simulink subsystem "Controller"  (R2020a)
settings: Solver=VariableStepAuto  StartTime=0.0  StopTime=10.0  RelTol=1e-3
undefined symbols (not defined in the file): N, PWM, TMAX, tmax, TMIN, tmin, Ts, Ui, Xi
libraries: mpclib x1
settings Model: Creator=Lamarre  LastModifiedBy=lamarre

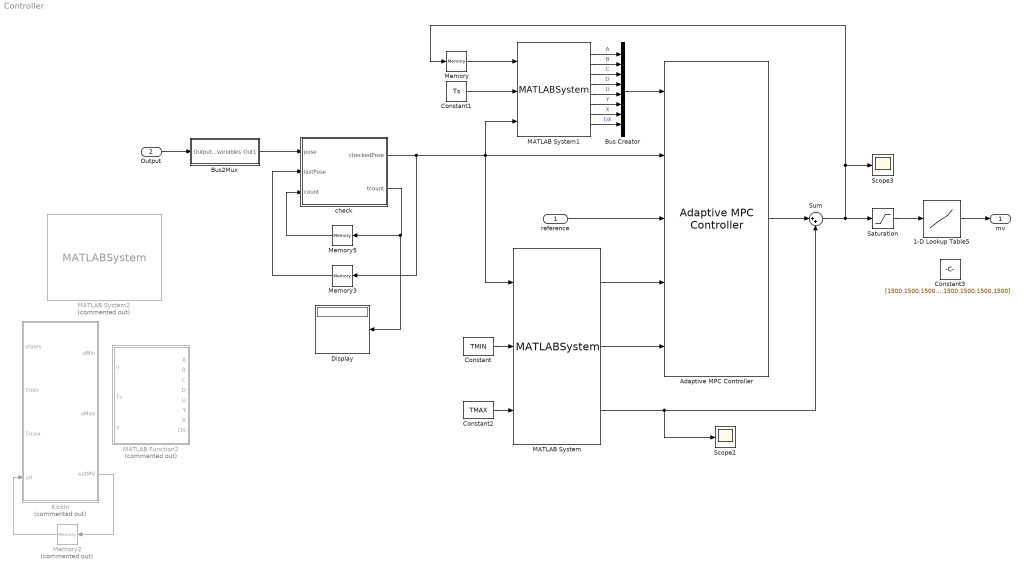
== system Controller ==
  reference : Inport
  Output : Inport  Port=2
  1-D Lookup Table5 : Lookup_n-D  NumberOfTableDimensions=1  BreakpointsForDimension1=N  Table=PWM  InterpMethod=Nearest  ExtrapMethod=Clip  InternalRulePriority=Speed  RndMeth=Simplest  InputSameDT=on
  Adaptive MPC Controller : mpclib/Adaptive MPC Controller  SCDEnableBlockLinearizationSpecification=on  mpcobj=mpcobj  enable_value=0  updateMPCinCallerWorkspace=on  md_inport=off  mv_inport=off  uref_inport=off  return_cost=off  return_mvseq=off  return_qpstatus=off  return_xseq=off  return_state=off  return_ovseq=off  state_inport=off  isltv_plant=off  umin_inport=on  umax_inport=on  ymin_inport=off  ymax_inport=off  cc_inport=off  ywt_inport=off  uwt_inport=off  duwt_inport=off  rhoeps_inport=off  pm_inport=off  MaximumP=10  HorizonChoice=FixedHorizon  BlockDataType=double  SampleTimeInherited=off  switch_inport=off
  Bus Creator : BusCreator  Inputs=8
  Bus2Mux : Subsystem
  Constant : Constant  Value=TMIN  VectorParams1D=off
  Constant1 : Constant  Value=Ts
  Constant2 : Constant  Value=TMAX
  Constant3 : Constant  Value=[1500,1500,1500,1500,1500,1500,1500,1500]
  Display : Display
  KickIn : MATLAB Function  Commented=on  TreatAsAtomicUnit=on  SystemSampleTime=Ts
  MATLAB Function2 : MATLAB Function  Commented=on  TreatAsAtomicUnit=on  SystemSampleTime=Ts
  MATLAB System : MATLABSystem  System=KickIn  SimulateUsing=Code generation
      mask Type: KickIn
      mask Display:
      | disp('KickIn');
      | port_label('input',1,'states');
      | port_label('input',2,'Tmin');
      | port_label('input',3,'Tmax');
      | port_label('output',1,'uMin');
      | port_label('output',2,'uMax');
      | port_label('output',3,'extMV');
  MATLAB System1 : MATLABSystem  System=TrimPlant  SimulateUsing=Code generation
      mask Type: TrimPlant
      mask Display:
      | disp('TrimPlant');
      | port_label('input',1,'u');
      | port_label('input',2,'Ts');
      | port_label('input',3,'y');
      | port_label('output',1,'A');
      | port_label('output',2,'B');
      | port_label('output',3,'C');
      | port_label('output',4,'D');
      | port_label('output',5,'U');
      | port_label('output',6,'Y');
      | port_label('output',7,'X');
      | port_label('output',8,'DX');
  MATLAB System2 : MATLABSystem  Commented=on  System=DiscontinuityCheck  SimulateUsing=Code generation
      mask Type: DiscontinuityCheck
      mask Display:
      | disp('DiscontinuityCheck');
      | port_label('input',1,'pose');
      | port_label('input',2,'IC');
      | port_label('output',1,'checkedPose');
      | port_label('output',2,'tour');
  Memory : Memory  InitialCondition=Ui
  Memory2 : Memory  Commented=on  InitialCondition=[0;0;0;0;-7.1;6.94;-7.49;7.65]
  Memory3 : Memory  InitialCondition=Xi
  Memory5 : Memory  InitialCondition=[0,0,0]
  Saturation : Saturate  UpperLimit=tmax  LowerLimit=tmin  LinearizeAsGain=off  ZeroCross=off
  Scope2 : Scope
  Scope3 : Scope
  Sum : Sum  Inputs=|++
  check : MATLAB Function  TreatAsAtomicUnit=on  SystemSampleTime=Ts
  mv : Outport
  wires:
  Sum/1 -> Memory/1, Scope3/1, Saturation/1
  Adaptive MPC Controller/1 -> Sum/1
  Bus Creator/1 -> Adaptive MPC Controller/1
  Memory/1 -> MATLAB System1/1
  Constant1/1 -> MATLAB System1/2
  reference/1 -> Adaptive MPC Controller/3
  Output/1 -> Bus2Mux/1(Output variables)
  Memory3/1 -> check/2(lastPose)
  Memory5/1 -> check/3(count)
  check/2(tcount) -> Memory5/1, Display/1
  KickIn/3(extMV) -> Memory2/1
  Memory2/1 -> KickIn/4(u0)
  MATLAB System/1 -> Adaptive MPC Controller/4
  MATLAB System/2 -> Adaptive MPC Controller/5
  MATLAB System/3 -> Sum/2, Scope2/1
  Constant2/1 -> MATLAB System/3
  Constant/1 -> MATLAB System/2
  MATLAB System1/1 -> Bus Creator/1  "A"
  MATLAB System1/2 -> Bus Creator/2  "B"
  MATLAB System1/3 -> Bus Creator/3  "C"
  MATLAB System1/4 -> Bus Creator/4  "D"
  MATLAB System1/5 -> Bus Creator/5  "U"
  MATLAB System1/6 -> Bus Creator/6  "Y"
  MATLAB System1/7 -> Bus Creator/7  "X"
  MATLAB System1/8 -> Bus Creator/8  "DX"
  Saturation/1 -> 1-D Lookup Table5/1
  check/1(checkedPose) -> Adaptive MPC Controller/2, MATLAB System1/3, MATLAB System/1, Memory3/1
  Bus2Mux/1(Out1) -> check/1(pose)
  1-D Lookup Table5/1 -> mv/1

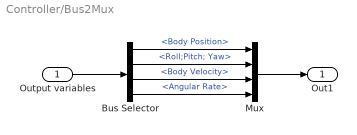
== system Controller/Bus2Mux ==
  Output variables : Inport
  Bus Selector : BusSelector  OutputSignals=Body Position,Roll;Pitch; Yaw,Body Velocity,Angular Rate
  Mux : Mux
  Out1 : Outport
  wires:
  Mux/1 -> Out1/1
  Output variables/1 -> Bus Selector/1
  Bus Selector/2 -> Mux/2  "<Roll;Pitch; Yaw>"
  Bus Selector/4 -> Mux/4  "<Angular Rate>"
  Bus Selector/1 -> Mux/1  "<Body Position>"
  Bus Selector/3 -> Mux/3  "<Body Velocity>"

== matlab function Controller/MATLAB Function2 ==
  data: u input; Ts input; y input; A output; B output; C output; D output; U output; Y output; X output; DX output
function [A,B,C,D,U,Y,X,DX] = TrimPlant(u,Ts,y)
% Lineariser le model dynamique

%x=[y(4:5,1);y(7:12,1)];
%x(5)=x(5)-.85;
tic;
[Ac, Bc, Cc, Dc]=AUVStateJacobianFcn(y,u);
% Generate discrete-time model

%  nx = size(Ac,1);
%  nu = size(Bc,2);
%cplant=ss(Ac,Bc,Cc,Dc);
%plant=c2d(cplant,Ts,'zoh');

nx = size(Ac,1);
nu = size(Bc,2);
M = expm([[Ac Bc]*Ts; zeros(nu,nu+nx)]);
A = M(1:nx,1:nx);
B = M(1:nx,nx+1:nx+nu);
C = Cc;
D = Dc;
 %xx=[X(4:5,1);X(7:12)];

% cplant=ss(Ac,Bc,Cc,Dc);
% plant=c2d(cplant,Ts,'zoh');
%plant=ss(A,B,C,D,Ts);

% Nominal conditions for discrete-time plant
U=u.';
Y=(Cc*y + Dc*u).';
X=y.';
DX=(A*y+B*u-y).';
toc;
end

== matlab function Controller/KickIn ==
  data: uMin output; uMax output; states input size=12; Tmin input; Tmax input; extMV output size=8; u0 input size=8
function [uMin,uMax,extMV] = KickIn(states,Tmin,Tmax,u0)

uMin=Tmin;
uMax=Tmax;

% Fonction objective.
fun = @(x)sum(abs(u0.'-x));

% Retrouver la matrice gravité et thruster
Aeq=ThrusterMatrix().';
Beq=Gravity(states).';

% Optimiser la commande pour la condition initial
op=optimoptions('fmincon','Algorithm','sqp','ConstraintTolerance',0.01,...
                'OptimalityTolerance',0.01);
            
extMV=-fmincon(fun,u0.',[],[],Aeq,Beq,[],[],[],op).';

% Calculer la nouvelle limite thruster
for i=1:size(extMV,1)
    if extMV(i)>0
        uMax(i)= uMax(i)-extMV(i);
    else
        uMin(i)= uMin(i)-extMV(i);
    end
end

== matlab function Controller/check ==
  data: pose input size=[12 1]; checkedPose output size=[12 1]; lastPose input size=[12 1]; count input size=3; tcount output
function[checkedPose,tcount]= discontinuityCheck(pose,lastPose,count)
           % Cette fonction vérifie et corrige au besoin la discontinuite
           % des angles de rotation.
           tcount=count;
           checkedPose=pose;
           
          for i=4:6 % compute roll pitch yaw
              
              % appliquer la discontinuté actuelle
               if tcount(i-3)>0
                   checkedPose(i)=(pose(i)+pi)+(pi*tcount(i-3));
               elseif tcount<0
                   checkedPose(i)=(pose(i)-pi)+(pi*tcount(i-3));
               end
               
               % calculer la différence entre 2 point
               delta=lastPose(i)-checkedPose(i);
              
               
               % Verifier la discontinuité de laxe
               if abs (delta)>=pi 
                   % Determiner le sens de la discontinuité
                   if delta >0 
                      % Ajouter un tour
                      tcount(i-3)=tcount(i-3)+1;
                      % Recaluler l'angle
                      checkedPose(i)=(pi+pose(i))+(pi*tcount(i-3));
                   else
                      % Soustraire un tour
                      tcount(i-3)=tcount(i-3)-1;
                      % Recaluler l'angle
                      checkedPose(i)=(pose(i)-pi)+(pi*tcount(i-3));
                   end
               end   
           end
end
